simulink model "QD2_DroneStack_PID_2021a"  (R2026a)
settings: Solver=ode1  StopTime=inf  FixedStep=1/1000  EnableMultiTasking=on
InitFcn:
  | Motor_Mapping_7_Inch
model workspace (MAT data in the model file):
  target_system = 1
undefined symbols (not defined in the file): _Commander, _Stabilizer, datetime, HIL, KT, lf, log_, log_QD2_, m, Motor_Matrix, n, qc_get_step_size, s, saved_data
libraries: quarc_library x106, simulink x26, simulink_extras x3
(part 5 of 5)

== matlab function QD2_DroneStack_PID_2021a/QDrone 2 DAQ/MATLAB Function ==
  data: mdl_time input; arm input; estop input; esc_problem input; cmd output; cmd_enable output; tele_enable output; esc_ready output; esc_timeout output; stop_mdl output; pre_state input; state output
function [cmd, cmd_enable, tele_enable, esc_ready, esc_timeout, stop_mdl, state] = esc_state_machine(mdl_time, arm, estop, esc_problem, pre_state)

persistent next_state_after_pause
persistent state_counter
persistent state_counter_after_pause
persistent esc_timeout_state

% Define state enumeration
STATE_INIT_WAIT = 0;
STATE_INIT_WAIT_EXTENDED = 1;
STATE_IDLE = 2;
STATE_CMD_BEEP = 3;
STATE_CMD_SET_DIRECTION = 4;
STATE_CMD_MOTOR = 5;
STATE_CMD_ZERO = 77;
STATE_CMD_DISABLED = 88;
STATE_EXIT = 99;

% Define state counter values
COUNT_STATE_INIT_MIN = 1000;
COUNT_STATE_INIT_MAX = 10000;
COUNT_STATE_IDLE = 1000;
COUNT_STATE_BEEP = 60;
%COUNT_STATE_BEEP = 1000;
COUNT_STATE_SET_DIRECTION = 120;
%COUNT_STATE_SET_DIRECTION = 500;
COUNT_STATE_DISABLE_BEEP = 1000;
COUNT_STATE_DISABLE_DIRECTION = 500;
COUNT_STATE_CMD_ZERO_PAUSE = 1000;


% Initialize persistent variables
if isempty(next_state_after_pause)
    next_state_after_pause = STATE_EXIT;
end
if isempty(state_counter)
    state_counter=COUNT_STATE_INIT_MIN;
end
if isempty(state_counter_after_pause)
    state_counter_after_pause = COUNT_STATE_IDLE;
end
if isempty(esc_timeout_state)
    esc_timeout_state = 0;
end


% Initialize output
state = STATE_INIT_WAIT;
cmd = [0,0,0,0];
tele_enable = 0;
cmd_enable = 0;
stop_mdl = 0;
esc_ready = 0;

% State Transition
% E-Stop superceeds all commands
if estop
    state = STATE_EXIT;
else
    switch pre_state
        % Initialization - send command zero and request telemetry
        case STATE_INIT_WAIT
            state_counter = state_counter - 1;
            if state_counter <= 0 
                % Go to next state
                state = STATE_INIT_WAIT_EXTENDED;
                state_counter = COUNT_STATE_INIT_MAX;
            else
                % Stay in current state
                state = pre_state;
            end
    
    
        % Extended initialization wait until ESC initialization completed
        case STATE_INIT_WAIT_EXTENDED
            state_counter = state_counter - 1;
            if state_counter <= 0
                % Max timeout reached, unrecoverable error condition, flag and
                % terminate.
                state = STATE_EXIT;
                esc_timeout_state = 1;
                
            else
                % Check if we are clear to proceed
                if esc_problem
                    % Stay in current state and keep waiting
                    state = pre_state;
                else
                    % Go to next state
                    state = STATE_CMD_ZERO;
                    state_counter = COUNT_STATE_CMD_ZERO_PAUSE;
                    next_state_after_pause = STATE_CMD_BEEP;
                    state_counter_after_pause = COUNT_STATE_BEEP;
                end
            end
    
        % Send Beep command
        case STATE_CMD_BEEP
            state_counter = state_counter - 1;
            if state_counter <= 0
                % Go to next state
                state = STATE_CMD_DISABLED;
                state_counter = COUNT_STATE_DISABLE_BEEP;
                next_state_after_pause = STATE_CMD_SET_DIRECTION;
                state_counter_after_pause = COUNT_STATE_SET_DIRECTION;
                % Alternately go directly to set direction
%                 state = STATE_CMD_SET_DIRECTION;
%                 state_counter = COUNT_STATE_SET_DIRECTION;
            else
                % Stay in current state
                state = pre_state;
            end
            
        % Set Direction
        case STATE_CMD_SET_DIRECTION
            state_counter = state_counter - 1;
            if state_counter <= 0
                % Go to next state
                state = STATE_CMD_DISABLED;
                state_counter = COUNT_STATE_DISABLE_DIRECTION;
                next_state_after_pause = STATE_IDLE;
                state_counter_after_pause = COUNT_STATE_IDLE;
            else
                % Stay in current state
                state = pre_state;
            end
    
        % Idle/Disarm state with telemetry enabled
        case STATE_IDLE
            if arm
                % Go to next state
                state = STATE_CMD_MOTOR;
            else
                % Stay and wait
                state = pre_state;
            end
            
        % Drive motor
        case STATE_CMD_MOTOR
            % Skip checking for telemetry fails after motor starts
%            if not(esc_problem)
                if not(arm)
                    % Go to next state
                    state = STATE_IDLE;
                else
                    % Stay in current state
                    state = pre_state;
                end
%             else
%                 % Not expecting this but flag it
%                 state = STATE_EXIT;
%                 esc_timeout_state = 1;
%             end
    
        % Pause with command disabled
        case STATE_CMD_DISABLED
            state_counter = state_counter - 1;
            if state_counter <= 0
                % Go to next state
                state = next_state_after_pause;
                state_counter = state_counter_after_pause;
            else
                % stay in current state
                state = pre_state;
            end
            
        % Generic pause state with command and telemetry enabled
        case STATE_CMD_ZERO
            state_counter = state_counter - 1;
            if state_counter <= 0
                % Got to next state
                state = next_state_after_pause;
                state_counter = state_counter_after_pause;
            else
                % Stay in current state
                state = pre_state;
            end 

        % Exit state
        case STATE_EXIT
            % Do nothing until model stop
            state = pre_state;
    end
end

% State Output
switch state
    % Command zero to initialize the ESC
    case STATE_INIT_WAIT
        cmd = [0, 0, 0, 0];
        tele_enable = 1;
        cmd_enable = 1;
        stop_mdl = 0;
        esc_ready = 0;

    % Extended wait during initialization to confirm all ESC are ready
    case STATE_INIT_WAIT_EXTENDED
        cmd = [0,0,0,0];
        tele_enable = 1;
        cmd_enable = 1;
        stop_mdl = 0;
        esc_ready = 0;

    % Send beep command
    case STATE_CMD_BEEP
        cmd = [1, 1, 1, 1]*3;
        %tele_enable = 0;
        % Old BLHeli firmware needs the telemetry bit set to accept beep
        % command
        tele_enable = 1;
        cmd_enable = 1;
        stop_mdl = 0;
        esc_ready = 0;

    % Set Direction
    case STATE_CMD_SET_DIRECTION
        % Normal - for old BLHeli firmware
        cmd = [20, 21, 21, 20];
        % Workaround - for new AM32 firmware - looks like a bug  
        %cmd = [21, 20, 20, 21];
        %cmd = [21, 21, 21, 21];
        %cmd = [20, 20, 20, 20];
        %tele_enable = 0;
        % old BLHeli firmware needs the telemetry bit set to accept set
        % direction command
        tele_enable = 1;
        cmd_enable = 1;
        stop_mdl = 0;
        esc_ready = 0;

    % Disarm command
    case STATE_IDLE
        cmd = [0,0,0,0];
        tele_enable = 0;
        cmd_enable = 1;
        stop_mdl = 0;
        esc_ready = 1;
        
    % Drive motors
    case STATE_CMD_MOTOR
        cmd = [48, 48, 48, 48];
        tele_enable = 1;
        cmd_enable = 1;
        stop_mdl = 0;
        esc_ready = 1;

    % Idle/disable state
    case STATE_CMD_DISABLED
        cmd = [0 0 0 0];
        tele_enable = 0;
        cmd_enable = 0;
        stop_mdl = 0;
        esc_ready = 0;

    % Generic Pause
    case STATE_CMD_ZERO
        cmd = [0,0,0,0];
        tele_enable = 1;
        cmd_enable = 1;
        stop_mdl = 0;
        esc_ready = 0;

    % Stop
    case STATE_EXIT
        cmd = [0,0,0,0];
        tele_enable = 0;
        cmd_enable = 1;
        stop_mdl = 1;
        esc_ready = 0;
end

% output esc_timeout variable
esc_timeout = esc_timeout_state;

== matlab function QD2_DroneStack_PID_2021a/QDrone 2 DAQ/Force to percentage Mapping ==
  data: V_Bat_Act input; Motor_Forces input; Duty_Cycle output; KT input
function Duty_Cycle = fcn(V_Bat_Act,Motor_Forces,KT)

B = KT(2)^2-4*KT(1)*(KT(3)-Motor_Forces)

invalid_signal = B < 0
B(invalid_signal) = 0

% Ranges from 1000-2000
Volt_CMD_Theo = -0.5*KT(2)/KT(1)+ sqrt(B)/(2*KT(1));

Duty_Cycle = Volt_CMD_Theo/V_Bat_Act;

== matlab function QD2_DroneStack_PID_2021a/COMMANDER (ANGLE MODE)/THROTTLE SWITCHBOX /Throttle Switchbox ==
  data: FSM_state input; sigmoid output
function sigmoid  = application_drone_throttle_switchbox(FSM_state)

% Application Drone: Throttle Switchbox
%
% Logic for switching between throttle commands from the controller 
%
% v2.0 - 5th october, 2018
%
% INPUTS:
% -------
% FSM_state = current state of the FSM------------------------------------------------------- (#)         [1]
% 
% OUTPUTS:
% --------
% sigmoid = an integer whose state determines how the heights are transformed---------------- (#)         [1]
% sigmoid = 1 - Command 0 throttle
% sigmoid = 2 - Sigmoid throttle up from 0 to the trim value
% sigmoid = 3 - Pass controller throttle straight through + trim value.
% sigmoid = 4 - Ignore controller throttle. Sigmoid it down to 0.
% sigmoid = 5 - Pass controller throttle straight through + trim value.


sigmoid = 0;
switch FSM_state
    case 1 % IDLE STATE
        sigmoid = 1;
    case 2 % ARM STATE
        sigmoid = 1;
    case 3 % TAKEOFF THROTTLE STATE
        sigmoid = 2;
    case 4 % TAKEOFF HEIGHT STATE
        sigmoid = 3;
    case 5 % FLIGHT STATE
        sigmoid = 3;
    case 6 % AUTOLAND STATE
        sigmoid = 5;
    case 7 % EMERGENCY STOP STATE
        sigmoid = 4;
    case 8 % EMERGENCY ABORT STATE
        sigmoid = 1;
    case 9 % DISABLE STATE
        sigmoid = 1;
end

== matlab function QD2_DroneStack_PID_2021a/HORIZON FRAME CONVERSION AND ESTIMATION/Pose Switchbox/MATLAB Function ==
  data: sigmoid_type input; enable output; x_des input; slow_lim input; fast_lim input; x_cur input; x_vel input; x_ref output; max_x_vel output; max_x_accel output; x_meas input
function [enable, x_ref, max_x_vel, max_x_accel] = fcn(sigmoid_type, x_des, slow_lim, fast_lim, x_cur, x_vel, x_meas)

% Note: Some of the cases below are identical. However, they are separated out 
% based on the states of the state machine for ease of modification in the future. 
% For example, states 4 and 5 are identical. However, if the user wants different 
% signmoid behaviour when taking off than when landing, these cases may not be the same. 

enable = 0;
x_ref = 0;
max_x_vel = 0;
max_x_accel = 0;

switch sigmoid_type
    case 1 % This is for the IDLE, ARM, E_ABORT, E_STOP and DISABLE states of the FSM
        enable = 1;
        x_ref = x_meas;
        max_x_vel = slow_lim(1);
        max_x_accel = slow_lim(2);

    case 2 % This is for the TAKEOFF THROTTLE state of the FSM
        enable = 1;
        x_ref = x_meas;
        max_x_vel = slow_lim(1);
        max_x_accel = slow_lim(2);

    case 3 % This is for the FLIGHT state of the FSM
        enable = 1;
        x_ref = x_des;
        max_x_vel = fast_lim(1);
        max_x_accel = fast_lim(2);

    case 4 % This is for the TAKEOFF HEIGHT state of the FSM
        enable = 1;
        x_ref = x_des;
        if (abs(x_cur - x_des) <= 0.02)
            max_x_vel = fast_lim(1);
            max_x_accel = fast_lim(2);
        else    
            max_x_vel = slow_lim(1);
            max_x_accel = slow_lim(2);
        end
    case 5 % This is for the AUTOLAND state of the FSM
        enable = 1;
        x_ref = x_des;
        if (abs(x_cur - x_des) <= 0.02)
            max_x_vel = fast_lim(1);
            max_x_accel = fast_lim(2);        
        else
            max_x_vel = slow_lim(1);
            max_x_accel = slow_lim(2);
        end
        
end

== matlab function QD2_DroneStack_PID_2021a/HORIZON FRAME CONVERSION AND ESTIMATION/Pose Switchbox/MATLAB Function1 ==
  data: sigmoid_type input; enable output; y_des input; slow_lim input; fast_lim input; y_cur input; y_vel input; y_ref output; max_y_vel output; max_y_accel output; y_meas input
function [enable, y_ref, max_y_vel, max_y_accel] = fcn(sigmoid_type, y_des, slow_lim, fast_lim, y_cur, y_vel, y_meas)

% Note: Some of the cases below are identical. However, they are separated out 
% based on the states of the state machine for ease of modification in the future. 
% For example, states 4 and 5 are identical. However, if the user wants different 
% signmoid behaviour when taking off than when landing, these cases may not be the same. 

enable = 0;
y_ref = 0;
max_y_vel = 0;
max_y_accel = 0;

switch sigmoid_type
    case 1 % This is for the IDLE, ARM, E_ABORT, E_STOP and DISABLE states of the FSM
        enable = 1;
        y_ref = y_meas;
        max_y_vel = slow_lim(1);
        max_y_accel = slow_lim(2);

    case 2 % This is for the TAKEOFF THROTTLE state of the FSM
        enable = 1;
        y_ref = y_meas;
        max_y_vel = slow_lim(1);
        max_y_accel = slow_lim(2);

    case 3 % This is for the FLIGHT state of the FSM
        enable = 1;
        y_ref = y_des;
        max_y_vel = fast_lim(1);
        max_y_accel = fast_lim(2);

    case 4 % This is for the TAKEOFF HEIGHT state of the FSM
        enable = 1;
        y_ref = y_des;
        if (abs(y_cur - y_des) <= 0.02)
            max_y_vel = fast_lim(1);
            max_y_accel = fast_lim(2);
        else    
            max_y_vel = slow_lim(1);
            max_y_accel = slow_lim(2);
        end
    case 5 % This is for the AUTOLAND state of the FSM
        enable = 1;
        y_ref = y_des;
        if (abs(y_cur - y_des) <= 0.02)
            max_y_vel = fast_lim(1);
            max_y_accel = fast_lim(2);        
        else
            max_y_vel = slow_lim(1);
            max_y_accel = slow_lim(2);
        end
        
end

== matlab function QD2_DroneStack_PID_2021a/HORIZON FRAME CONVERSION AND ESTIMATION/Pose Switchbox/MATLAB Function2 ==
  data: sigmoid_type input; enable output; height_des input; slow_lim input; fast_lim input; height_cur input; height_vel input; height_ref output; max_height_vel output; max_height_accel output
function [enable, height_ref, max_height_vel, max_height_accel] = fcn(sigmoid_type, height_des, slow_lim, fast_lim, height_cur, height_vel)

% Note: Some of the cases below are identical. However, they are separated out 
% based on the states of the state machine for ease of modification in the future. 
% For example, states 4 and 5 are identical. However, if the user wants different 
% signmoid behaviour when taking off than when landing, these cases may not be the same. 

enable = 0;
height_ref = 0;
max_height_vel = 0;
max_height_accel = 0;

switch sigmoid_type
    case 1 % This is for the IDLE, ARM, E_ABORT, E_STOP and DISABLE states of the FSM
        enable = 0;
        height_ref = 0;
        max_height_vel = 0;
        max_height_accel = 0;

    case 2 % This is for the TAKEOFF THROTTLE state of the FSM
        enable = 0;
        height_ref = 0;
        max_height_vel = 0;
        max_height_accel = 0;

    case 3 % This is for the FLIGHT state of the FSM 
        enable = 1;
        height_ref = height_des;
        max_height_vel = fast_lim(1);
        max_height_accel = fast_lim(2);

    case 4 % This is for the TAKEOFF HEIGHT state of the FSM
        enable = 1;
        height_ref = height_des;
        if (height_vel < 0)||(abs(height_cur - height_des) <= 0.1)||(height_des <= height_cur)
            max_height_vel = fast_lim(1);
            max_height_accel = fast_lim(2);
        else    
            max_height_vel = slow_lim(1);
            max_height_accel = slow_lim(2);
        end
    case 5 % This is for the AUTOLAND state of the FSM
        enable = 1;
        height_ref = 0;
        if height_vel >= 0
            max_height_vel = fast_lim(1);
            max_height_accel = fast_lim(2);        
        else
            max_height_vel = slow_lim(1);
            max_height_accel = slow_lim(2);
        end
        
end
